simulink model "LQG Simulink"  (R2016a)
settings: Solver=VariableStepAuto  StartTime=0.0  StopTime=10.0  RelTol=1e-3
values from neighbouring files (symbols this model uses):
  a = [0.9801  0.0003 -0.0980  0.0038 ... (first row only)    [LQG Controller.m]
  b = [-0.0001  0.0058; 0.0296  0.0153; 0.0012 -0.0908; 0.0015  0.0008]    [LQG Controller.m]
  c = [1 0 0 0;0 0 0 1]    [LQG Controller.m]
  d = [0 0; 0 0]    [LQG Controller.m]
  Kr = lqr(a,b,Q,R)    [LQG Controller.m]
undefined symbols (not defined in the file or in its folder): Ke
settings Model: Creator=engrh  LastModifiedBy=engrh

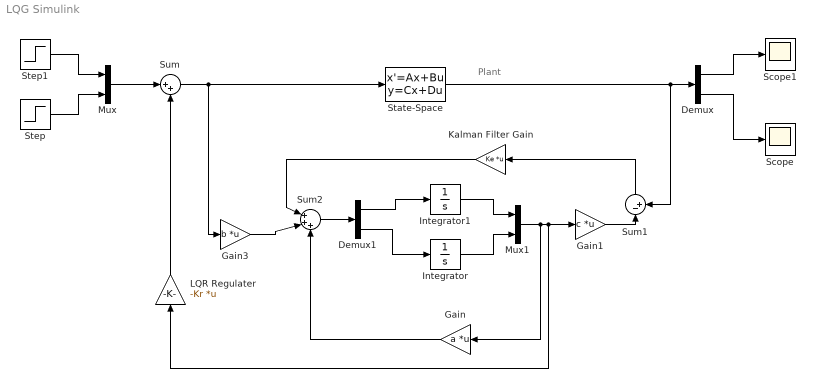
== system LQG Simulink ==
  note: Plant
  Demux : Demux  Outputs=2
  Demux1 : Demux  Outputs=2
  Gain : Gain  Gain=a  Multiplication=Matrix(K*u)
  Gain1 : Gain  Gain=c  Multiplication=Matrix(K*u)
  Gain3 : Gain  Gain=b  Multiplication=Matrix(K*u)
  Integrator : Integrator
  Integrator1 : Integrator
  Kalman Filter Gain : Gain  Gain=Ke  Multiplication=Matrix(K*u)
  LQR Regulater : Gain  Gain=-Kr  Multiplication=Matrix(K*u)
  Mux : Mux  Inputs=2
  Mux1 : Mux  Inputs=2
  Scope : Scope
  Scope1 : Scope
  State-Space : StateSpace  A=a  B=b  C=c  D=d  X0=0
  Step : Step  SampleTime=0
  Step1 : Step  SampleTime=0
  Sum : Sum  Inputs=|++
  Sum1 : Sum  Inputs=|-+
  Sum2 : Sum  Inputs=|+++
  wires:
  Sum/1 -> Gain3/1, State-Space/1
  Mux/1 -> Sum/1
  Step1/1 -> Mux/1
  Step/1 -> Mux/2
  Demux/1 -> Scope1/1
  Demux/2 -> Scope/1
  Mux1/1 -> Gain/1, Gain1/1, LQR Regulater/1
  Demux1/1 -> Integrator1/1
  Sum2/1 -> Demux1/1
  Demux1/2 -> Integrator/1
  Integrator1/1 -> Mux1/1
  Integrator/1 -> Mux1/2
  Gain1/1 -> Sum1/1
  State-Space/1 -> Sum1/2, Demux/1
  Sum1/1 -> Kalman Filter Gain/1
  Kalman Filter Gain/1 -> Sum2/1
  Gain/1 -> Sum2/3
  Gain3/1 -> Sum2/2
  LQR Regulater/1 -> Sum/2
